simulink model "Exp1"  (Simulink 7.7)
settings: Solver=ode23s  StartTime=0.0  StopTime=20  RelTol=1e-3
undefined symbols (not defined in the file): RL, Rsh
libraries: powerlib x27, simulink x1
settings Model: Creator=Meikandasivam  LastModifiedBy=Meikandasivam

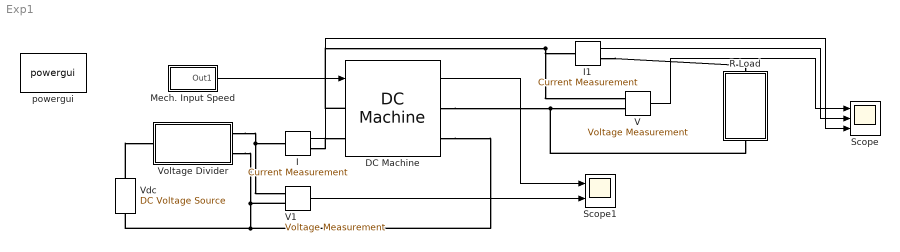
== system Exp1 ==
  DC Machine : powerlib/Machines/DC Machine  SystemSampleTime=-1  PresetModel=01: 5HP 240V 1750RPM Field:300V  MechanicalLoad=Speed w  FieldType=Wound  ShowDetailedParameters=on  RLa=[2.581 0.028]  RLf=[281.3 156]  Laf=0.9483  MachineConstant=Torque constant (N.m/A)  Ke=1.8  Kt=1.8  J=0.02215  Bm=0.002953  Tf=0.5161  w0=1  Ifinit=1  TsPowergui=0  TsBlock=-1
      settings: AttributesFormatString=\n
  I : powerlib/Measurements/Current Measurement  SystemSampleTime=-1  PhasorSimulation=off  OutputType=Complex  PSBequivalent=0
  I1 : powerlib/Measurements/Current Measurement  SystemSampleTime=-1  PhasorSimulation=off  OutputType=Complex  PSBequivalent=0
  Mech. Input Speed : Subsystem
  R Load : Subsystem
  Scope : Scope  NumInputPorts=3
      settings: YMin=0.235~0.00149354~-5  YMax=0.2525~0.00165076~5
  Scope1 : Scope  NumInputPorts=2
      settings: YMin=0~0  YMax=175~400  SaveName=ScopeData2
  V : powerlib/Measurements/Voltage Measurement  SystemSampleTime=-1  PhasorSimulation=off  OutputType=Complex  PSBequivalent=0
  V1 : powerlib/Measurements/Voltage Measurement  SystemSampleTime=-1  PhasorSimulation=off  OutputType=Complex  PSBequivalent=0
  Vdc : powerlib/Electrical Sources/DC Voltage Source  SystemSampleTime=-1  Amplitude=450  Measurements=None
  Voltage Divider : Subsystem
  powergui : powerlib/powergui  Priority=1  SystemSampleTime=-1  SimulationMode=Continuous  SampleTime=50e-6  frequency=60  SPID=off  DisableSnubberDevices=off  DisableRonSwitches=off  DisableVfSwitches=off  SwTol=0  Interpol=off  DisplayEquations=off  FunctionMessages=off  frequencyindice=0  Pbase=100e6  ErrMax=1e-4  Iterations=50  UnitsV=kV  UnitsW=MW  echomessages=off  HookPort=off  EnableUseOfTLC=off  x0status=blocks  RestoreLinks=warning  ResistiveCurrentMeasurement=off  Ylog=off  Xlog=on  ShowGrid=off  save=off  variable=ZData  ZoomFFT=off  StartTime=0.0  cycles=1  DisplayStyle=1  FreqAxis=off  MaxFrequency=1000  frequencyindicesteady=1  display=off  methode=off
  wires:
  Mech. Input Speed/1(Out1) -> DC Machine/1
  DC Machine/1 -> Scope1/1
  V1/1 -> Scope1/2
  V/1 -> Scope/1
  I1/1 -> Scope/2
  I/1 -> Scope/3
  connections:
  V1/LConn2 -- DC Machine/RConn2 -- Vdc/LConn1 -- Voltage Divider/RConn2
  I/RConn1 -- DC Machine/LConn2
  R Load/RConn1 -- DC Machine/RConn1 -- V/LConn2
  DC Machine/LConn1 -- V/LConn1 -- I1/LConn1
  Vdc/RConn1 -- Voltage Divider/LConn1
  Voltage Divider/RConn1 -- I/LConn1 -- V1/LConn1
  I1/RConn1 -- R Load/LConn1

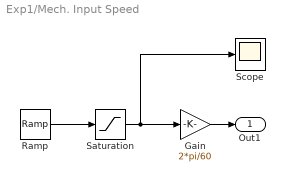
== system Exp1/Mech. Input Speed ==
  Gain : Gain  Gain=2*pi/60
  Ramp : simulink/Sources/Ramp  SystemSampleTime=-1  slope=1770  start=0  X0=0
  Saturation : Saturate  UpperLimit=1500  LowerLimit=0
  Scope : Scope
  Out1 : Outport
  wires:
  Ramp/1 -> Saturation/1
  Saturation/1 -> Scope/1, Gain/1
  Gain/1 -> Out1/1

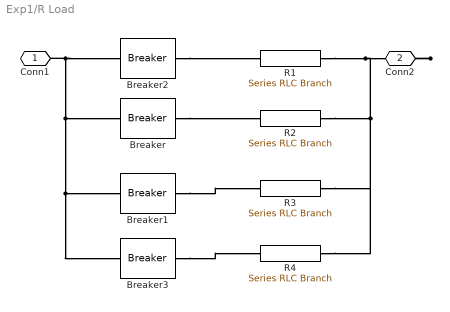
== system Exp1/R Load ==
  Breaker : powerlib/Elements/Breaker  SystemSampleTime=-1  BreakerResistance=0.01  InitialState=0  SnubberResistance=1e6  SnubberCapacitance=inf  SwitchingTimes=[ 18 19 ]  External=off  Measurements=None  MoreParameters=off  NoBreakLoop=off
  Breaker1 : powerlib/Elements/Breaker  SystemSampleTime=-1  BreakerResistance=0.01  InitialState=0  SnubberResistance=1e6  SnubberCapacitance=inf  SwitchingTimes=[ 19 20 ]  External=off  Measurements=Branch current  MoreParameters=off  NoBreakLoop=off
  Breaker2 : powerlib/Elements/Breaker  SystemSampleTime=-1  BreakerResistance=0.01  InitialState=0  SnubberResistance=1e6  SnubberCapacitance=inf  SwitchingTimes=[ 17 18]  External=off  Measurements=None  MoreParameters=off  NoBreakLoop=off
  Breaker3 : powerlib/Elements/Breaker  SystemSampleTime=-1  BreakerResistance=0.01  InitialState=0  SnubberResistance=1e6  SnubberCapacitance=inf  SwitchingTimes=[ 20 21 ]  External=off  Measurements=None  MoreParameters=off  NoBreakLoop=off
  R{1..4} (4 alike) : powerlib/Elements/Series RLC Branch  PhysicalDomain=powersysdomain  SubClassName=unknown  LeftPortType=p1  RightPortType=p1  LConnTagsString=__new0  RConnTagsString=__new0  BranchType=R  Resistance=RL  Inductance=1e-3  SetiL0=off  InitialCurrent=0  Capacitance=1e-6  Setx0=off  InitialVoltage=0  Measurements=None
  Conn1 : PMIOPort  Port=1  Side=Left
  Conn2 : PMIOPort  Port=2  Side=Right
  connections:
  Conn1/RConn1 -- Breaker2/LConn1 -- Breaker/LConn1 -- Breaker1/LConn1 -- Breaker3/LConn1
  Breaker/RConn1 -- R2/LConn1
  Breaker1/RConn1 -- R3/LConn1
  Breaker2/RConn1 -- R1/LConn1
  Breaker3/RConn1 -- R4/LConn1
  Conn2/RConn1 -- R1/RConn1 -- R2/RConn1 -- R3/RConn1 -- R4/RConn1

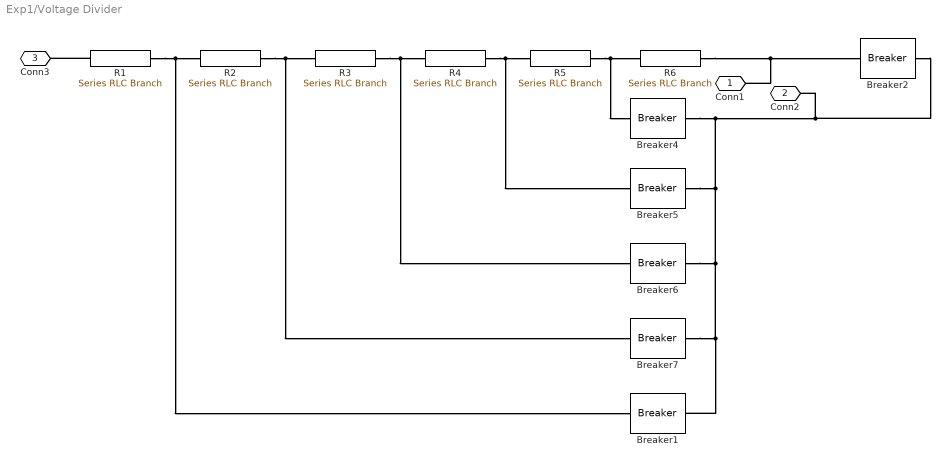
== system Exp1/Voltage Divider ==
  Breaker1 : powerlib/Elements/Breaker  SystemSampleTime=-1  BreakerResistance=0.01  InitialState=0  SnubberResistance=1e6  SnubberCapacitance=inf  SwitchingTimes=[ 4 6 ]  External=off  Measurements=Branch voltage and current  MoreParameters=off  NoBreakLoop=off
  Breaker2 : powerlib/Elements/Breaker  SystemSampleTime=-1  BreakerResistance=0.01  InitialState=0  SnubberResistance=1e6  SnubberCapacitance=inf  SwitchingTimes=[ 14 16]  External=off  Measurements=Branch voltage and current  MoreParameters=off  NoBreakLoop=off
  Breaker4 : powerlib/Elements/Breaker  SystemSampleTime=-1  BreakerResistance=0.01  InitialState=0  SnubberResistance=1e6  SnubberCapacitance=inf  SwitchingTimes=[ 12 14]  External=off  Measurements=Branch voltage and current  MoreParameters=off  NoBreakLoop=off
  Breaker5 : powerlib/Elements/Breaker  SystemSampleTime=-1  BreakerResistance=0.01  InitialState=0  SnubberResistance=1e6  SnubberCapacitance=inf  SwitchingTimes=[ 10 12 ]  External=off  Measurements=None  MoreParameters=off  NoBreakLoop=off
  Breaker6 : powerlib/Elements/Breaker  SystemSampleTime=-1  BreakerResistance=0.01  InitialState=0  SnubberResistance=1e6  SnubberCapacitance=inf  SwitchingTimes=[ 8 10 ]  External=off  Measurements=None  MoreParameters=off  NoBreakLoop=off
  Breaker7 : powerlib/Elements/Breaker  SystemSampleTime=-1  BreakerResistance=0.01  InitialState=0  SnubberResistance=1e6  SnubberCapacitance=inf  SwitchingTimes=[ 6 8 ]  External=off  Measurements=None  MoreParameters=off  NoBreakLoop=off
  R{1..6} (6 alike) : powerlib/Elements/Series RLC Branch  PhysicalDomain=powersysdomain  SubClassName=unknown  LeftPortType=p1  RightPortType=p1  LConnTagsString=__new0  RConnTagsString=__new0  BranchType=R  Resistance=Rsh  Inductance=1e-3  SetiL0=off  InitialCurrent=0  Capacitance=1e-6  Setx0=off  InitialVoltage=0  Measurements=None
  Conn1 : PMIOPort  Port=1  Side=Left
  Conn2 : PMIOPort  Port=2  Side=Right
  Conn3 : PMIOPort  Port=3  Side=Right
  connections:
  R1/RConn1 -- Breaker1/LConn1 -- R2/LConn1
  Breaker1/RConn1 -- Breaker5/RConn1 -- Breaker4/RConn1 -- Conn2/RConn1 -- Breaker2/RConn1 -- Breaker6/RConn1 -- Breaker7/RConn1
  R5/RConn1 -- Breaker4/LConn1 -- R6/LConn1
  R4/RConn1 -- Breaker5/LConn1 -- R5/LConn1
  R3/RConn1 -- Breaker6/LConn1 -- R4/LConn1
  R2/RConn1 -- Breaker7/LConn1 -- R3/LConn1
  R1/LConn1 -- Conn3/RConn1
  R6/RConn1 -- Conn1/RConn1 -- Breaker2/LConn1
